simulink model "massive_mimo_simulink"  (R2025a)
settings: Solver=VariableStepAuto  StartTime=0.0  StopTime=10.0  RelTol=1e-3
undefined symbols (not defined in the file or in its folder): doppler
libraries: commchan3 x2, commdigbbndpm3 x2, commsink2 x1, commrandsrc3 x1
settings Model: Creator=yyash  LastModifiedBy=yyash

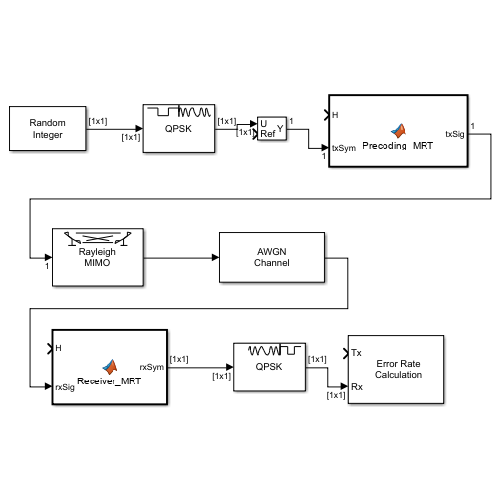
[thumbnail: Simulink's stored preview of the top-level diagram]
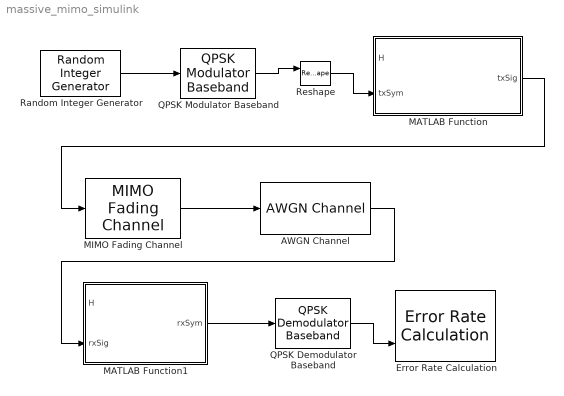
== system massive_mimo_simulink ==
  AWGN Channel : commchan3/AWGN Channel  LegacyMode=off  NoiseMethod="Signal to noise ratio  (SNR)"  noiseMode="Signal to noise ratio  (SNR)"  EbNo=10  EsNo=10  SNR=10  BitsPerSymbol=1  SignalPower=1  SpecifySymbolPeriod=off  SamplesPerSymbol=1  SymbolPeriod=1  VarianceSource=Parameter  Variance=1  RandomStream=Global stream  Seed=67  SimulateUsing=Code generation
  Error Rate Calculation : commsink2/Error Rate Calculation  N=0  st_delay=0  cp_mode=Entire frame  subframe=[]  PMode=Workspace  WsName=ErrorVec  RsMode2=off  stop=off  numErr=100  maxBits=1e6
  MATLAB Function : MATLAB Function  TreatAsAtomicUnit=on
  MATLAB Function1 : MATLAB Function  TreatAsAtomicUnit=on
  MIMO Fading Channel : commchan3/MIMO Fading Channel  InheritSampleRate=on  SampleRate=1  PathDelays=0  AveragePathGains=0  NormalizePathGains=on  FadingDistribution=Rayleigh  KFactor=3  DirectPathDopplerShift=0  DirectPathInitialPhase=0  MaximumDopplerShift=0.001  DopplerSpectrum=doppler('Jakes')  SpatialCorrelationSpecification=None  SpatialCorrelationMatrix=[1 0 0 0; 0 1 0 0; 0 0 1 0; 0 0 0 1]  NumTransmitAntennas=2  NumReceiveAntennas=2  TransmitCorrelationMatrix=[1 0; 0 1]  ReceiveCorrelationMatrix=[1 0; 0 1]  AntennaSelection=Off  NormalizeChannelOutputs=on  PathGainsOutputPort=off  SimulateUsing=Interpreted execution  FadingTechnique=Filtered Gaussian noise  NumSinusoids=48  InitialTimeSource=Property  InitialTime=0  RandomStream=mt19937ar with seed  Seed=73  Visualization=Off  AntennaPairsToDisplay=[ 1, 1 ]  PathsForDopplerDisplay=1  SamplesToDisplay=25%
  QPSK Demodulator Baseband : commdigbbndpm3/QPSK Demodulator Baseband  OutType=Integer  DecType=Hard decision  VarSource=Dialog  Variance=1  Dec=Gray  Ph=pi/4  outDtype1=Inherit via internal rule  outDtype2=Inherit via internal rule  derotateFactorWordLen=16  derotateFactorDataTypeStr=Inherit: Same word length as input  derotateFactorLastDataTypeStr=Inherit: Same word length as input
      settings: LibrarySourceBlock=|
      | commhdldigbbndpm/QPSK
      | Demodulator
      | Baseband
  QPSK Modulator Baseband : commdigbbndpm3/QPSK Modulator Baseband  InType=Integer  Enc=Gray  Ph=pi/4  outDtype=double  outWordLen=16  outUDDataType=sfix(16)  outFracLenMode=Best precision  outFracLen=15  outDataTypeStr=double  outLastDataTypeStr=double
  Random Integer Generator : commrandsrc3/Random Integer Generator  SetSize=4  SeedSource=Auto  Seed=0  SampleTime=1  SamplesPerFrame=1  OutputDataType=double  SimulateUsing=Interpreted execution
  Reshape : Reshape  OutputDimensionality=Derive from reference input port
  wires:
  Random Integer Generator/1 -> QPSK Modulator Baseband/1
  QPSK Modulator Baseband/1 -> Reshape/1
  Reshape/1 -> MATLAB Function/2(txSym)
  MATLAB Function/1(txSig) -> MIMO Fading Channel/1
  MIMO Fading Channel/1 -> AWGN Channel/1
  AWGN Channel/1 -> MATLAB Function1/2(rxSig)
  MATLAB Function1/1(rxSym) -> QPSK Demodulator Baseband/1
  QPSK Demodulator Baseband/1 -> Error Rate Calculation/2

== matlab function massive_mimo_simulink/MATLAB Function ==
  data: H input; txSig output; txSym input
function txSig = Precoding_MRT(H, txSym)
% H: Nr×Nt channel matrix
% txSym: Nt×1 transmit symbol vector
% txSig: Nt×1 precoded transmit vector
W = H';                     % MRT precoder
W = W / norm(W,'fro');      % Normalize power
txSig = W * txSym;
end

== matlab function massive_mimo_simulink/MATLAB Function1 ==
  data: H input; rxSym output; rxSig input
function rxSym = Receiver_MRT(H, rxSig)
% rxSig: received Nr×1 vector
W = H';                     % same MRT weights
W = W / norm(W,'fro');
rxSym = W' * rxSig;         % combine
end
